simulink model "ex7"  (Simulink 8.7)
settings: Solver=VariableStepDiscrete  StartTime=0.0  StopTime=SimulationTime  RelTol=1e-3
libraries: commutil2 x4, commsink2 x2, commfilt2 x2, commdigbbndpm3 x2, commchan3 x1, commrandsrc2 x1
settings Model: Creator=Zhouwt  LastModifiedBy=Zhouwt
settings DataIOCC: SignalLoggingSaveFormat=ModelDataLogs
settings OptimizationCC: InitFltsAndDblsToZero=on
settings DebuggingCC: SaveWithParameterizedLinksMsg=none  SignalResolutionControl=TryResolveAllWithWarning  SolverPrmCheckMsg=warning  MultiTaskDSMMsg=warning  MultiTaskCondExecSysMsg=none
settings GRTTargetCC: TargetFcnLib=ansi_tfl_tmw.mat  GeneratePreprocessorConditionals=Use local settings  CombineOutputUpdateFcns=off  GRTInterface=on

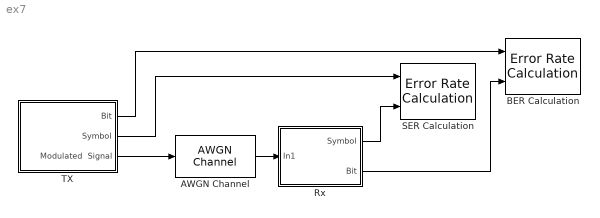
== system ex7 ==
  AWGN Channel : commchan3/AWGN Channel  InputProcessing=Inherited (this choice will be removed - see release notes)  seed=123456  noiseMode="Signal to noise ratio  (SNR)"  EbNodB=10  EsNodB=10  SNRdB=SNR  bitsPerSym=1  Ps=1  Tsym=1  variance=1
  BER Calculation : commsink2/Error Rate Calculation  N=0  st_delay=0  cp_mode=Entire frame  subframe=[]  PMode=Workspace  WsName=BER  RsMode2=off  stop=off  numErr=100  maxBits=1e6
  Rx : Subsystem
  SER Calculation : commsink2/Error Rate Calculation  N=0  st_delay=0  cp_mode=Entire frame  subframe=[]  PMode=Workspace  WsName=SER  RsMode2=off  stop=off  numErr=100  maxBits=1e6
  TX : Subsystem
  wires:
  TX/3(Modulated  Signal) -> AWGN Channel/1
  AWGN Channel/1 -> Rx/1(In1)
  TX/2(Symbol) -> SER Calculation/1
  Rx/1(Symbol) -> SER Calculation/2
  TX/1(Bit) -> BER Calculation/1
  Rx/2(Bit) -> BER Calculation/2

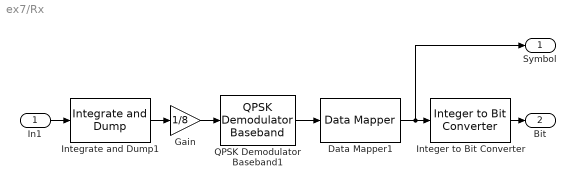
== system ex7/Rx ==
  In1 : Inport
  Data Mapper1 : commutil2/Data Mapper  MapMode=Gray to Binary  M=4  MapVec=[0 1 3 2 7 6 4 5]
  Gain : Gain  Gain=1/8
  Integer to Bit Converter : commutil2/Integer to Bit Converter  nbits=2  signedInputValues=Unsigned  bitOrder=MSB first  outDtype=Inherit via internal rule
  Integrate and Dump1 : commfilt2/Integrate and Dump  obssamples=8  offsetsamples=0  nodump=off  roundingMode=Floor  overflowMode=off  outputDataTypeStr=Inherit: Same as accumulator  outputLastDataTypeStr=Inherit: Same as accumulator
  QPSK Demodulator Baseband1 : commdigbbndpm3/QPSK Demodulator Baseband  OutType=Integer  DecType=Hard decision  VarSource=Dialog  Variance=1  Dec=Gray  Ph=0  outDtype1=Inherit via internal rule  outDtype2=Inherit via internal rule  derotateFactorWordLen=16  derotateFactorDataTypeStr=Inherit: Same word length as input  derotateFactorLastDataTypeStr=Inherit: Same word length as input
  Symbol : Outport
  Bit : Outport  Port=2
  wires:
  Integrate and Dump1/1 -> Gain/1
  Integer to Bit Converter/1 -> Bit/1
  Data Mapper1/1 -> Integer to Bit Converter/1, Symbol/1
  In1/1 -> Integrate and Dump1/1
  Gain/1 -> QPSK Demodulator Baseband1/1
  QPSK Demodulator Baseband1/1 -> Data Mapper1/1

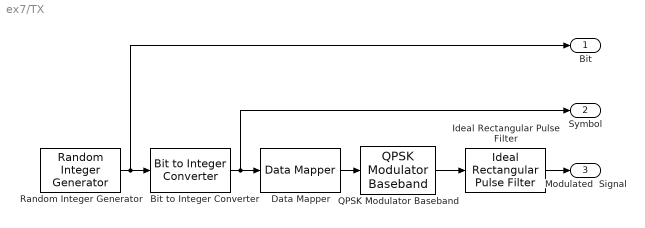
== system ex7/TX ==
  Bit to Integer Converter : commutil2/Bit to Integer Converter  nbits=2  bitOrder=MSB first  signedOutputValues=Unsigned  outDtype=Inherit via internal rule  outDtypeSigned=Inherit via internal rule
  Data Mapper : commutil2/Data Mapper  MapMode=Binary to Gray  M=4  MapVec=[0 1 3 2 7 6 4 5]
  Ideal Rectangular Pulse Filter : commfilt2/Ideal Rectangular Pulse Filter  pulseLen=8  pulseDelay=0  InputProcessing=Columns as channels (frame based)  RateOptions=Enforce single-rate processing  sampMode=Mute  normCheck=off  normMode=Energy per pulse  filterGain=1  saveAsFlag=0  roundingMode=Floor  overflowMode=off  firstCoeffDataTypeStr=Inherit: Same word length as input  firstCoeffMin=[]  firstCoeffMax=[]  firstCoeffLastDataTypeStr=Inherit: Same word length as input  outputDataTypeStr=Inherit: Same as accumulator  outputMin=[]  outputMax=[]  outputLastDataTypeStr=Inherit: Same as accumulator
  QPSK Modulator Baseband : commdigbbndpm3/QPSK Modulator Baseband  InType=Integer  Enc=Gray  Ph=0  outDtype=double  outWordLen=16  outUDDataType=sfix(16)  outFracLenMode=Best precision  outFracLen=15  outDataTypeStr=double  outLastDataTypeStr=double
  Random Integer Generator : commrandsrc2/Random Integer Generator  mul=2  seed=37  Ts=1/400000  frameBased=on  sampPerFrame=400000  orient=off  outDataType=double
  Bit : Outport
  Symbol : Outport  Port=2
  Modulated  Signal : Outport  Port=3
  wires:
  Ideal Rectangular Pulse Filter/1 -> Modulated  Signal/1
  Random Integer Generator/1 -> Bit to Integer Converter/1, Bit/1
  Bit to Integer Converter/1 -> Data Mapper/1, Symbol/1
  QPSK Modulator Baseband/1 -> Ideal Rectangular Pulse Filter/1
  Data Mapper/1 -> QPSK Modulator Baseband/1
